simulink model "BusSelector2"  (R2017b)
settings: Solver=FixedStepDiscrete  StartTime=0.0  StopTime=10.0  FixedStep=0.200000  RelTol=1e-3
PreLoadFcn:
  | % Bus object: subBus
  | clear elems;
  | elems(1) = Simulink.BusElement;
  | elems(1).Name = 'chirp';
  | elems(1).Dimensions = 2;
  | elems(1).DimensionsMode = 'Fixed';
  | elems(1).DataType = 'double';
  | elems(1).SampleTime = -1;
  | elems(1).Complexity = 'real';
  | elems(1).Min = [];
  | elems(1).Max = [];
  | elems(1).DocUnits = '';
  | elems(1).Description = '';
  | 
  | elems(2) = Simulink.BusElement;
  | elems(2).Name = 'sine';
  | elems(2).Dimensions = 3;
  | elems(2).DimensionsMode = 'Fixed';
  | elems(2).DataType = 'int32';
  | elems(2).SampleTime = -1;
  | elems(2).Complexity = 'real';
  | elems(2).Min = [];
  | elems(2).Max = [];
  | elems(2).DocUnits = '';
  | elems(2).Description = '';
  | 
  | subBus = Simulink.Bus;
  | subBus.HeaderFile = '';
  | subBus.Description = '';
  | subBus.DataScope = 'Auto';
  | subBus.Alignment = -1;
  | subBus.Elements = elems;
  | clear elems;
  | assignin('base','subBus', subBus);
  | 
  | % Bus object: topBus
  | clear elems;
  | elems(1) = Simulink.BusElement;
  | elems(1).Name = 'subSignal';
  | elems(1).Dimensions = 1;
  | elems(1).DimensionsMode = 'Fixed';
  | elems(1).DataType = 'Bus: subBus';
  | elems(1).SampleTime = -1;
  | elems(1).Complexity = 'real';
  | elems(1).Min = [];
  | elems(1).Max = [];
  | elems(1).DocUnits = '';
  | elems(1).Description = '';
  | 
  | elems(2) = Simulink.BusElement;
  | elems(2).Name = 'step';
  | elems(2).Dimensions = 4;
  | elems(2).DimensionsMode = 'Fixed';
  | elems(2).DataType = 'boolean';
  | elems(2).SampleTime = -1;
  | elems(2).Complexity = 'real';
  | elems(2).Min = [];
  | elems(2).Max = [];
  | elems(2).DocUnits = '';
  | elems(2).Description = '';
  | 
  | topBus = Simulink.Bus;
  | topBus.HeaderFile = '';
  | topBus.Description = '';
  | topBus.DataScope = 'Auto';
  | topBus.Alignment = -1;
  | topBus.Elements = elems;
  | clear elems;
  | assignin('base','topBus', topBus);
settings Model: Creator=The MathWorks, Inc.  LastModifiedBy=hbourbou
settings DataIOCC: SaveFormat=Structure
settings OptimizationCC: LifeSpan=inf
settings DebuggingCC: SFExecutionAtInitializationDiag=none
settings HardwareCC: ProdBitPerSizeT=32  ProdBitPerPtrDiffT=32  ProdWordSize=32  ProdHWDeviceType=Specified
settings CodeAppCC: StateflowObjectComments=on
settings ConfigComp: CovMetricSettings=dswe

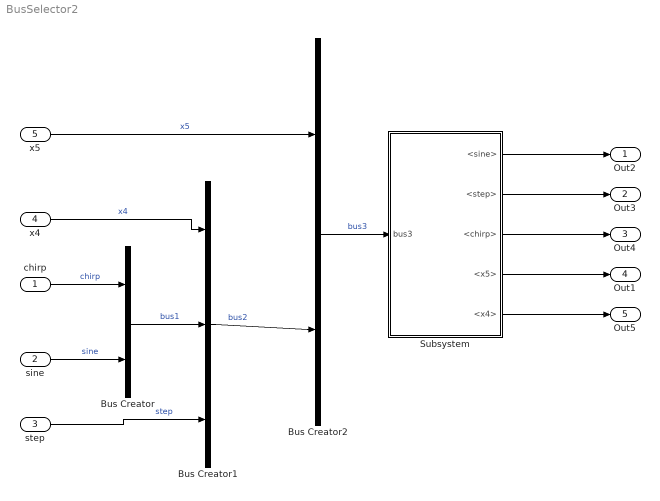
== system BusSelector2 ==
  chirp : Inport  OutDataTypeStr=double
  sine : Inport  Port=2  OutDataTypeStr=int32  PortDimensions=3
  step : Inport  Port=3  OutDataTypeStr=boolean  PortDimensions=4
  x4 : Inport  Port=4  OutDataTypeStr=boolean  PortDimensions=5
  x5 : Inport  Port=5  OutDataTypeStr=boolean  PortDimensions=5
  Bus Creator1 : BusCreator  Inputs=3
      settings: AttributesFormatString=NestedBus
  Bus Creator2 : BusCreator  Inputs=2
      settings: AttributesFormatString=NestedBus
  Bus Creator : BusCreator  Inputs=2
      settings: AttributesFormatString=SubBus
  Subsystem : Subsystem
  Out2 : Outport
  Out3 : Outport  Port=2
  Out4 : Outport  Port=3
  Out1 : Outport  Port=4
  Out5 : Outport  Port=5
  wires:
  chirp/1 -> Bus Creator/1  "chirp"
  Bus Creator/1 -> Bus Creator1/2  "bus1"
  sine/1 -> Bus Creator/2  "sine"
  step/1 -> Bus Creator1/3  "step"
  Bus Creator1/1 -> Bus Creator2/2  "bus2"
  x4/1 -> Bus Creator1/1  "x4"
  x5/1 -> Bus Creator2/1  "x5"
  Bus Creator2/1 -> Subsystem/1(bus3)  "bus3"
  Subsystem/1(<sine>) -> Out2/1
  Subsystem/2(<step>) -> Out3/1
  Subsystem/3(<chirp>) -> Out4/1
  Subsystem/4(<x5>) -> Out1/1
  Subsystem/5(<x4>) -> Out5/1

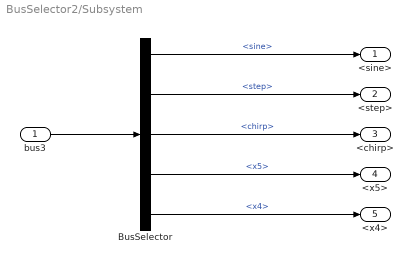
== system BusSelector2/Subsystem ==
  bus3 : Inport
  BusSelector : BusSelector  OutputSignals=bus2.bus1.sine,bus2.step,bus2.bus1.chirp,x5,bus2.x4
      settings: AttributesFormatString=Bus Selector
  <sine> : Outport
  <step> : Outport  Port=2
  <chirp> : Outport  Port=3
  <x5> : Outport  Port=4
  <x4> : Outport  Port=5
  wires:
  BusSelector/1 -> <sine>/1  "<sine>"
  BusSelector/5 -> <x4>/1  "<x4>"
  BusSelector/3 -> <chirp>/1  "<chirp>"
  bus3/1 -> BusSelector/1
  BusSelector/2 -> <step>/1  "<step>"
  BusSelector/4 -> <x5>/1  "<x5>"
